simulink model "mj_gettingStarted"  (R2022b)
settings: Solver=VariableStepAuto  StartTime=0.0  StopTime=inf  RelTol=1e-3
undefined symbols (not defined in the file): gray
libraries: mjLib x4
settings Model: Creator=vmano  LastModifiedBy=vmano
settings ModelReferenceCC: EnableRefExpFcnMdlSchedulingChecks=on
settings SFSimCC: SimTargetLang=C++

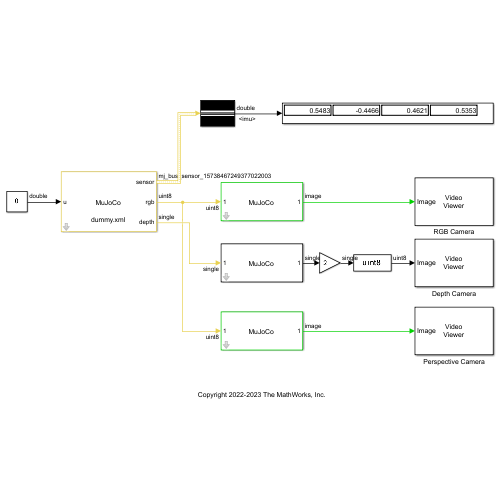
[thumbnail: Simulink's stored preview of the top-level diagram]
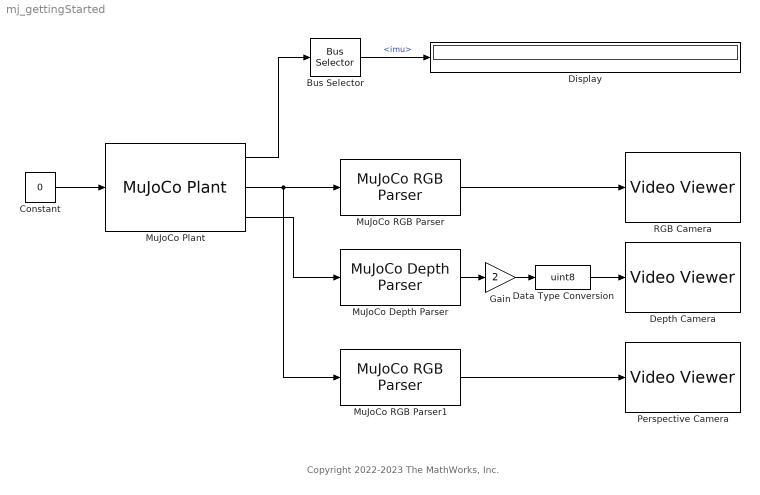
== system mj_gettingStarted ==
  note: Copyright 2022-2023 The MathWorks, Inc.
  Bus Selector : BusSelector  OutputSignals=imu
  Constant : Constant  Value=0
  Data Type Conversion : DataTypeConversion  OutDataTypeStr=uint8  SaturateOnIntegerOverflow=off  RndMeth=Floor
  Depth Camera : VideoViewer  colormapValue=gray(256)  FigPos=[998.6 1520.4 418.4 464.8]
  Display : Display
  Gain : Gain  Gain=2
  MuJoCo Depth Parser : mjLib/MuJoCo Depth Parser  inputBusType=mj_bus_rgb_3624495926710663437  selectedCamera=camera  imageRows=480  imageCols=640  startingIndex=307201  endingIndex=614400
      settings: SourceProductName=MuJoCo Simulator
  MuJoCo Plant : mjLib/MuJoCo Plant  controlBus=[]  sensorBus=mj_bus_sensor_7979902499018342666  controlLength=[]  sensorLength=[]  rgbLength=[]  depthLength=[]  sampleTime=0.005  xmlFileRel=dummy.xml  xmlFile=C:\work\GITLAB\mujoco-simulink-blockset\blocks\dummy.xml  renderingType=Global  vsync=off  visualFPS=60  zoomLevel=1  znear=0.059256  zfar=296.2816  cameraSampleTime=0.020  rgbOutOption=on  depthOutOption=on  controlInterfaceType=Vector
      settings: SourceProductName=MuJoCo Simulator
  MuJoCo RGB Parser : mjLib/MuJoCo RGB Parser  inputBusType=mj_bus_rgb_3624495926710663437  selectedCamera=camera  imageRows=480  imageCols=640  startingIndex=921601  endingIndex=1843200
      settings: SourceProductName=MuJoCo Simulator
  MuJoCo RGB Parser1 : mjLib/MuJoCo RGB Parser  inputBusType=mj_bus_rgb_3624495926710663437  selectedCamera=PerspectiveCamera  imageRows=480  imageCols=640  startingIndex=1  endingIndex=921600
      settings: SourceProductName=MuJoCo Simulator
  Perspective Camera : VideoViewer  colormapValue=gray(256)  FigPos=[1018.6 930.8 418.4 304]
  RGB Camera : VideoViewer  FigPos=[1443.4 1478 418.4 304]
  wires:
  MuJoCo Plant/2 -> MuJoCo RGB Parser1/1, MuJoCo RGB Parser/1
  MuJoCo Plant/3 -> MuJoCo Depth Parser/1
  MuJoCo Plant/1 -> Bus Selector/1
  Bus Selector/1 -> Display/1  "<imu>"
  MuJoCo RGB Parser/1 -> RGB Camera/1
  MuJoCo Depth Parser/1 -> Gain/1
  Constant/1 -> MuJoCo Plant/1
  Data Type Conversion/1 -> Depth Camera/1
  Gain/1 -> Data Type Conversion/1
  MuJoCo RGB Parser1/1 -> Perspective Camera/1
